simulink model "rtmc"  (R2014b)
settings: Solver=ode45  StartTime=0.0  StopTime=10.0  RelTol=1e-3
settings Model: Creator=mkatliar  LastModifiedBy=mkatliar

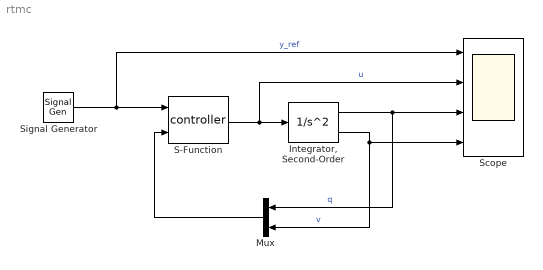
== system rtmc ==
  "Integrator, Second-Order" : SecondOrderIntegrator
  Mux : Mux  Inputs=2
  S-Function : S-Function  FunctionName=controller  EnableBusSupport=off
  Scope : Scope  NumInputPorts=4
      settings: TimeRange=10  YMin=-1~-1~0~-9.28709771634953e-17  YMax=1~1~2~0.4  ScrollMode=on
  Signal Generator : SignalGenerator
  wires:
  S-Function/1 -> Scope/2, "Integrator, Second-Order"/1  "u"
  "Integrator, Second-Order"/1 -> Mux/1, Scope/3  "q"
  Signal Generator/1 -> S-Function/1, Scope/1  "y_ref"
  "Integrator, Second-Order"/2 -> Mux/2, Scope/4  "v"
  Mux/1 -> S-Function/2
